simulink model "mbus_debus_bus"  (Simulink 6.1)
settings: Solver=ode5  StartTime=0.0  StopTime=30  RelTol=1e-3
PreLoadFcn:
  | load dbus_debus_bus.mat
settings Model: Creator=The MathWorks Inc.  LastModifiedBy=mshakeri  ExtModeAutoUpdateStatusClock=off  StrictBusMsg=ErrorLevel1  ProdHWDeviceType=Specified
settings DataIOCC: SignalLoggingName=logsOut
settings OptimizationCC: InlineParams=on
settings DebuggingCC: CheckExecutionContextPreStartOutputMsg=on  CheckExecutionContextRuntimeOutputMsg=on
settings HardwareCC: ProdHWDeviceType=Specified  TargetHWDeviceType=32-bit Generic  ProdEqTarget=off
settings ModelReferenceCC: UpdateModelReferenceTargets=IfOutOfDate
settings RTWCC: ProcessScript=grt_make_rtw_hook

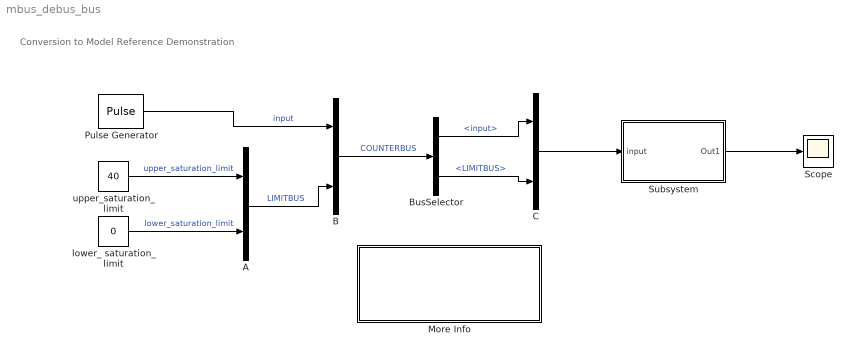
== system mbus_debus_bus ==
  note: Conversion to Model Reference Demonstration
  A : BusCreator  Inputs=2
  B : BusCreator  Inputs=2
  BusSelector : BusSelector  OutputSignals=input,LIMITBUS
  C : BusCreator  Inputs=2
  More Info : Subsystem
      settings: OpenFcn=mdlref_conversionscript
      mask Display: disp('Double click here \nfor a step-by-step\ntutorial on this model')
  Pulse Generator : DiscretePulseGenerator  Amplitude=int32(1)  SampleTime=0.1
  Scope : Scope
      settings: TimeRange=30  YMax=50  DataFormat=Array
  Subsystem : Subsystem  TreatAsAtomicUnit=on
  lower_ saturation_ limit : Constant  Value=0  OutDataTypeMode=int32  SampleTime=0.1
  upper_saturation_limit : Constant  Value=40  OutDataTypeMode=int32  SampleTime=0.1
  wires:
  upper_saturation_limit/1 -> A/1  "upper_saturation_limit"
  lower_ saturation_ limit/1 -> A/2  "lower_saturation_limit"
  A/1 -> B/2  "LIMITBUS"
  B/1 -> BusSelector/1  "COUNTERBUS"
  Pulse Generator/1 -> B/1  "input"
  BusSelector/1 -> C/1  "<input>"
  BusSelector/2 -> C/2  "<LIMITBUS>"
  C/1 -> Subsystem/1(" input")
  Subsystem/1(Out1) -> Scope/1

== system mbus_debus_bus/More Info ==
  note: This demonstration shows how signals may be grouped and ungrouped while
      | retaining their names.  In this demonstration, 5 signals are created and labelled
      | appropriately.  These signals are then mux'd together to create a bus of signals.
      | This bus of signals is then fed into the Bus Selector block.  Inside of the Bus
      | Selector block, the Pulse and Chirp signals are chosen to be output from the
      | original signal bus.
      |
      | It is possible to place a nest signal buses and then still retrieve the original signal
      | with its label.
  note: Bus Block Demonstration

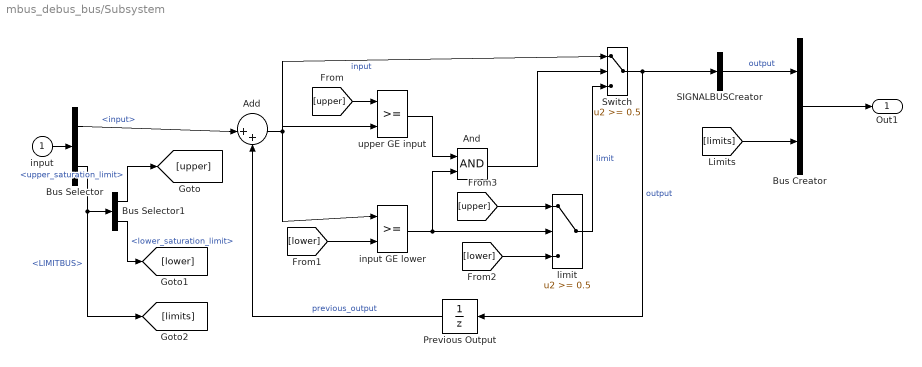
== system mbus_debus_bus/Subsystem ==
  " input" : Inport  Port=1  LatchInput=off
  " input GE lower" : RelationalOperator  Priority=1  InputSameDT=on
      settings: AttributesFormatString=\n
  " limit" : Switch  Threshold=0.5  SaturateOnIntegerOverflow=on  InputSameDT=on
  Add : Sum  Inputs=|++  OutScaling=2^-10
  And : Logic
  Bus Creator : BusCreator  Inputs=2
  Bus Selector : BusSelector  OutputSignals=input,LIMITBUS
  Bus Selector1 : BusSelector  OutputSignals=upper_saturation_limit,lower_saturation_limit
  Previous Output : UnitDelay  Orientation=left  SampleTime=-1
  SIGNALBUSCreator : BusCreator  Inputs=1
  Switch : Switch  Threshold=0.5  SaturateOnIntegerOverflow=on  InputSameDT=on
  upper GE input : RelationalOperator  Priority=0  InputSameDT=on
      settings: AttributesFormatString=\n
  Out1 : Outport
  wires:
  SIGNALBUSCreator/1 -> Bus Creator/1  "output"
  [limits] -> Bus Creator/2
  Bus Creator/1 -> Out1/1
  Bus Selector1/2 -> [lower]  "<lower_saturation_limit>"
  Bus Selector1/1 -> [upper]  "<upper_saturation_limit>"
  Bus Selector/1 -> Add/1  "<input>"
  Bus Selector/2 -> Bus Selector1/1, [limits]  "<LIMITBUS>"
  " input"/1 -> Bus Selector/1
  Add/1 -> " input GE lower"/1, upper GE input/2, Switch/1  "input"
  And/1 -> Switch/2
  " input GE lower"/1 -> And/2, " limit"/2
  [lower] -> " input GE lower"/2
  [upper] -> upper GE input/1
  [lower] -> " limit"/3
  Previous Output/1 -> Add/2  "previous_output"
  upper GE input/1 -> And/1
  " limit"/1 -> Switch/3  "limit"
  Switch/1 -> Previous Output/1, SIGNALBUSCreator/1  "output"
  [upper] -> " limit"/1
